simulink library "VLSGains"  (R2022b)
settings: Solver=VariableStepAuto  StartTime=0.0  StopTime=10.0  RelTol=1e-3
values from neighbouring files (symbols this model uses):
  VLSGainsConfig = struct('sample_rate_in_hertz', sample_rate_in_hertz,                              'frame_size', frame_size,                              'rgain_SILENT_GAIN', rgain_SILENT_GAIN,                              'granularity', internal_granularity,                              'numGains', numGains)    [VLSGainsInit.m]
  VLSGainsTune = load(VLSGainsTuneFileName)    [VLSGainsInit.m]
undefined symbols (not defined in the file or in its folder): Row
libraries: TuneVar x36, TOP x18, FeaturePath x2
(part 1 of 2)
settings Model: Creator=ud1041536  LastModifiedBy=jr1038734
settings SolverCC: AlgebraicLoopSolver=TrustRegion
settings DebuggingCC: UnconnectedInputMsg=warning  UnconnectedOutputMsg=warning  UnconnectedLineMsg=warning  SFMachineParentedDataDiag=warning
settings ModelReferenceCC: EnableRefExpFcnMdlSchedulingChecks=on

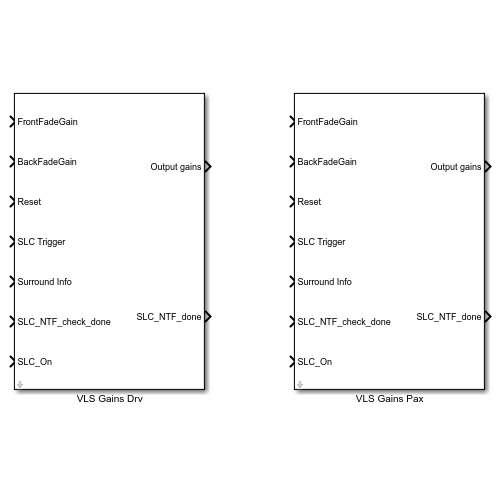
[thumbnail: Simulink's stored preview of the top-level diagram]
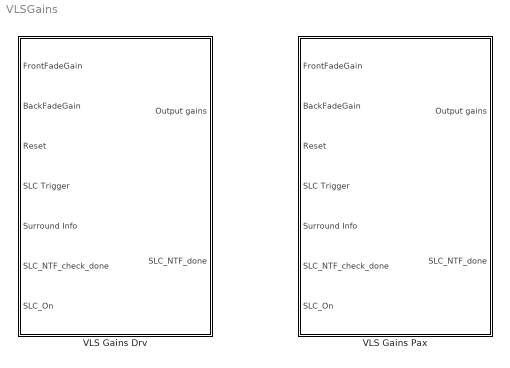
== system VLSGains ==
  VLS Gains Drv : Subsystem  mask(VLS Gains){configStruct=VLSGainsConfig, tuneStruct=VLSGainsTune, FeatureName=DrvGains}
      mask prompts: configStruct "Config struct name:"; tuneStruct "Tune struct name:"; FeatureName "FeaturePath name:"
      mask init:
      | VLSGainsMaskInit(gcbh, FeatureName);
      mask TypeOptions FeatureName: FeaturePath/FeatureName
  VLS Gains Pax : Subsystem  mask(VLS Gains){configStruct=VLSGainsConfig, tuneStruct=VLSGainsTune, FeatureName=PaxGains}
      mask prompts: configStruct "Config struct name:"; tuneStruct "Tune struct name:"; FeatureName "FeaturePath name:"
      mask init:
      | VLSGainsMaskInit(gcbh, FeatureName);
      mask TypeOptions FeatureName: FeaturePath/FeatureName

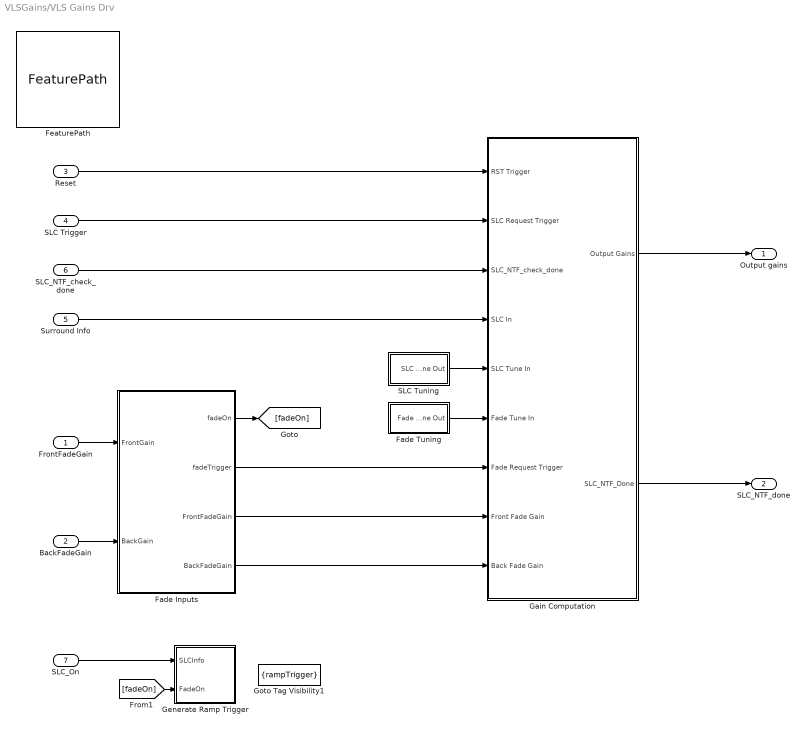
== system VLSGains/VLS Gains Drv ==
  FrontFadeGain : Inport
  BackFadeGain : Inport  Port=2
  Reset : Inport  Port=3
  SLC Trigger : Inport  Port=4
  Surround Info : Inport  Port=5
  SLC_NTF_check_done : Inport  Port=6
  SLC_On : Inport  Port=7
  Fade Inputs : Subsystem
  Fade Tuning : Subsystem
  FeaturePath : FeaturePath/FeaturePath  FeatureName=DrvGains  IsGroup=off  GroupNumber=-1  IsModule=off  TriggerInit=[125 254 250 371]
      settings: SourceProductName=Bose Talaria
  Gain Computation : Subsystem
  Generate Ramp Trigger : Subsystem
  Goto Tag Visibility1 : GotoTagVisibility  GotoTag=rampTrigger
  SLC Tuning : Subsystem
  Output gains : Outport  VectorParamsAs1DForOutWhenUnconnected=off
  SLC_NTF_done : Outport  Port=2  VectorParamsAs1DForOutWhenUnconnected=off
  wires:
  FrontFadeGain/1 -> Fade Inputs/1(FrontGain)
  Gain Computation/2(SLC_NTF_Done) -> SLC_NTF_done/1
  BackFadeGain/1 -> Fade Inputs/2(BackGain)
  SLC_NTF_check_done/1 -> Gain Computation/3(SLC_NTF_check_done)
  Reset/1 -> Gain Computation/1(RST Trigger)
  SLC Trigger/1 -> Gain Computation/2(SLC Request Trigger)
  Fade Tuning/1(Fade Tune Out) -> Gain Computation/6(Fade Tune In)
  Fade Inputs/3(FrontFadeGain) -> Gain Computation/8(Front Fade Gain)
  Gain Computation/1(Output Gains) -> Output gains/1
  Surround Info/1 -> Gain Computation/4(SLC In)
  Fade Inputs/4(BackFadeGain) -> Gain Computation/9(Back Fade Gain)
  SLC Tuning/1(SLC Tune Out) -> Gain Computation/5(SLC Tune In)
  Fade Inputs/2(fadeTrigger) -> Gain Computation/7(Fade Request Trigger)
  [fadeOn] -> Generate Ramp Trigger/2(FadeOn)
  SLC_On/1 -> Generate Ramp Trigger/1(SLCInfo)
  Fade Inputs/1(fadeOn) -> [fadeOn]

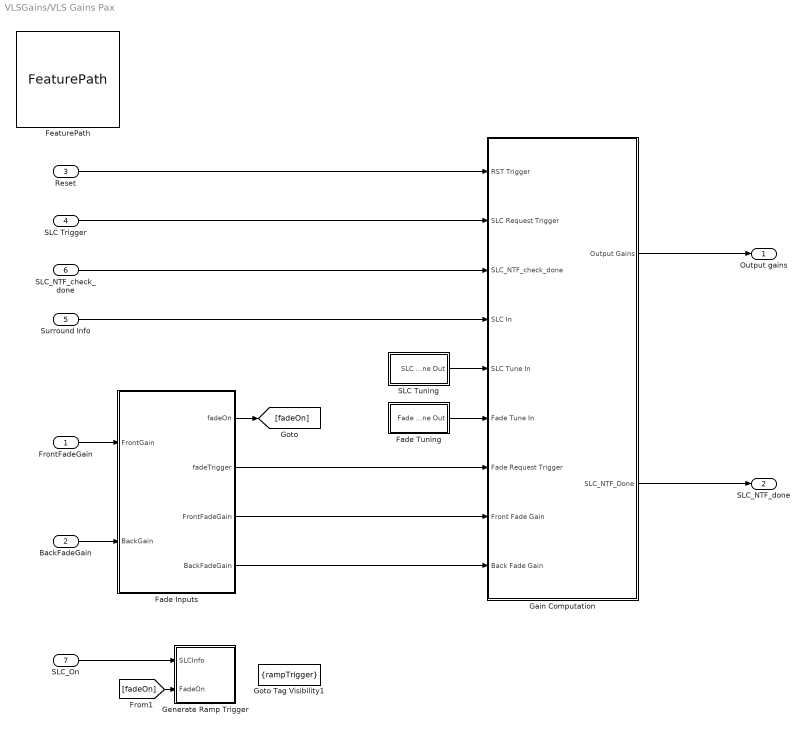
== system VLSGains/VLS Gains Pax ==
  FrontFadeGain : Inport
  BackFadeGain : Inport  Port=2
  Reset : Inport  Port=3
  SLC Trigger : Inport  Port=4
  Surround Info : Inport  Port=5
  SLC_NTF_check_done : Inport  Port=6
  SLC_On : Inport  Port=7
  Fade Inputs : Subsystem
  Fade Tuning : Subsystem
  FeaturePath : FeaturePath/FeaturePath  FeatureName=PaxGains  IsGroup=off  GroupNumber=-1  IsModule=off  TriggerInit=[125 254 250 371]
      settings: SourceProductName=Bose Talaria
  Gain Computation : Subsystem
  Generate Ramp Trigger : Subsystem
  Goto Tag Visibility1 : GotoTagVisibility  GotoTag=rampTrigger
  SLC Tuning : Subsystem
  Output gains : Outport  VectorParamsAs1DForOutWhenUnconnected=off
  SLC_NTF_done : Outport  Port=2  VectorParamsAs1DForOutWhenUnconnected=off
  wires:
  FrontFadeGain/1 -> Fade Inputs/1(FrontGain)
  Gain Computation/2(SLC_NTF_Done) -> SLC_NTF_done/1
  BackFadeGain/1 -> Fade Inputs/2(BackGain)
  SLC_NTF_check_done/1 -> Gain Computation/3(SLC_NTF_check_done)
  Reset/1 -> Gain Computation/1(RST Trigger)
  SLC Trigger/1 -> Gain Computation/2(SLC Request Trigger)
  Fade Tuning/1(Fade Tune Out) -> Gain Computation/6(Fade Tune In)
  Fade Inputs/3(FrontFadeGain) -> Gain Computation/8(Front Fade Gain)
  Gain Computation/1(Output Gains) -> Output gains/1
  Surround Info/1 -> Gain Computation/4(SLC In)
  Fade Inputs/4(BackFadeGain) -> Gain Computation/9(Back Fade Gain)
  SLC Tuning/1(SLC Tune Out) -> Gain Computation/5(SLC Tune In)
  Fade Inputs/2(fadeTrigger) -> Gain Computation/7(Fade Request Trigger)
  [fadeOn] -> Generate Ramp Trigger/2(FadeOn)
  SLC_On/1 -> Generate Ramp Trigger/1(SLCInfo)
  Fade Inputs/1(fadeOn) -> [fadeOn]

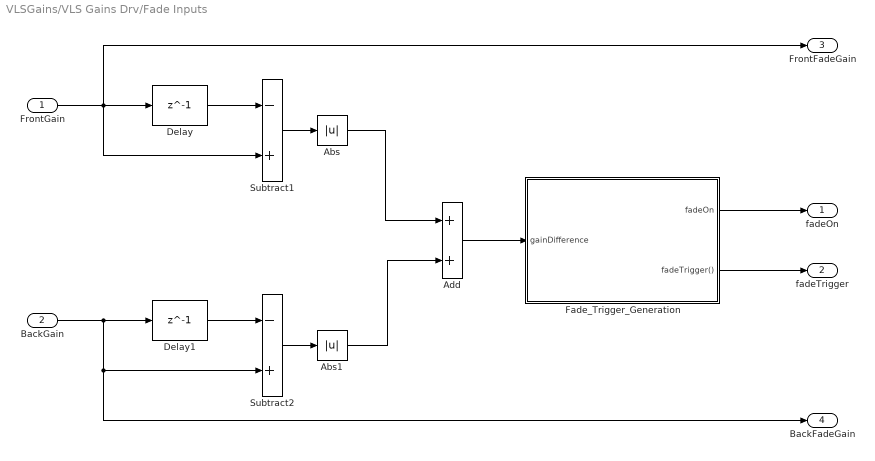
== system VLSGains/VLS Gains Drv/Fade Inputs ==
  FrontGain : Inport
  BackGain : Inport  Port=2
  Abs : Abs  SaturateOnIntegerOverflow=off
  Abs1 : Abs  SaturateOnIntegerOverflow=off
  Add : Sum
  Delay : Delay  DelayLength=1
  Delay1 : Delay  DelayLength=1
  Fade_Trigger_Generation : MATLAB Function  TreatAsAtomicUnit=on
  Subtract1 : Sum  Inputs=-+
  Subtract2 : Sum  Inputs=-+
  fadeOn : Outport
  fadeTrigger : Outport  Port=2  VectorParamsAs1DForOutWhenUnconnected=off
  FrontFadeGain : Outport  Port=3  VectorParamsAs1DForOutWhenUnconnected=off
  BackFadeGain : Outport  Port=4  VectorParamsAs1DForOutWhenUnconnected=off
  wires:
  BackGain/1 -> BackFadeGain/1, Subtract2/2, Delay1/1
  Abs1/1 -> Add/2
  Abs/1 -> Add/1
  Subtract2/1 -> Abs1/1
  Subtract1/1 -> Abs/1
  FrontGain/1 -> Subtract1/2, FrontFadeGain/1, Delay/1
  Delay/1 -> Subtract1/1
  Delay1/1 -> Subtract2/1
  Add/1 -> Fade_Trigger_Generation/1(gainDifference)
  Fade_Trigger_Generation/2(fadeTrigger()) -> fadeTrigger/1
  Fade_Trigger_Generation/1(fadeOn) -> fadeOn/1

== system VLSGains/VLS Gains Drv/Fade Tuning ==
  Backward Downmix Max : Subsystem  Description=This is the fraction of downmixing that occurs when 100% fade (back) is reached.
  Backward Downmix Threshold : Subsystem  Description=This is the fraction of fade (back) at which downmixing of premix coefficients starts.
  Downmix Weights : Subsystem  Description=These are the mixing weights at fader extreme when downmix_max is set to 1.
  Forward Downmix Threshold : Subsystem  Description=This is the fraction of fade (front) at which downmixing of premix coefficients starts.
  Foward Downmix Max : Subsystem  Description=This is the fraction of downmixing that occurs when 100% fade (front) is reached.
  Bus Element Out : Outport  VectorParamsAs1DForOutWhenUnconnected=off  PortName=Fade Tune Out  Element=Forward Downmix Threshold
  Bus Element Out1 : Outport  VectorParamsAs1DForOutWhenUnconnected=off  PortName=Fade Tune Out  Element=Forward Downmix Max
  Bus Element Out2 : Outport  VectorParamsAs1DForOutWhenUnconnected=off  PortName=Fade Tune Out  Element=Backward Downmix Threshold
  Bus Element Out3 : Outport  VectorParamsAs1DForOutWhenUnconnected=off  PortName=Fade Tune Out  Element=Backward Downmix Max
  Bus Element Out4 : Outport  VectorParamsAs1DForOutWhenUnconnected=off  PortName=Fade Tune Out  Element=Downmix Weights
  wires:
  Downmix Weights/1(Out1) -> Bus Element Out4/1
  Backward Downmix Threshold/1(Out1) -> Bus Element Out2/1
  Backward Downmix Max/1(Out1) -> Bus Element Out3/1
  Foward Downmix Max/1(Out1) -> Bus Element Out1/1
  Forward Downmix Threshold/1(Out1) -> Bus Element Out/1

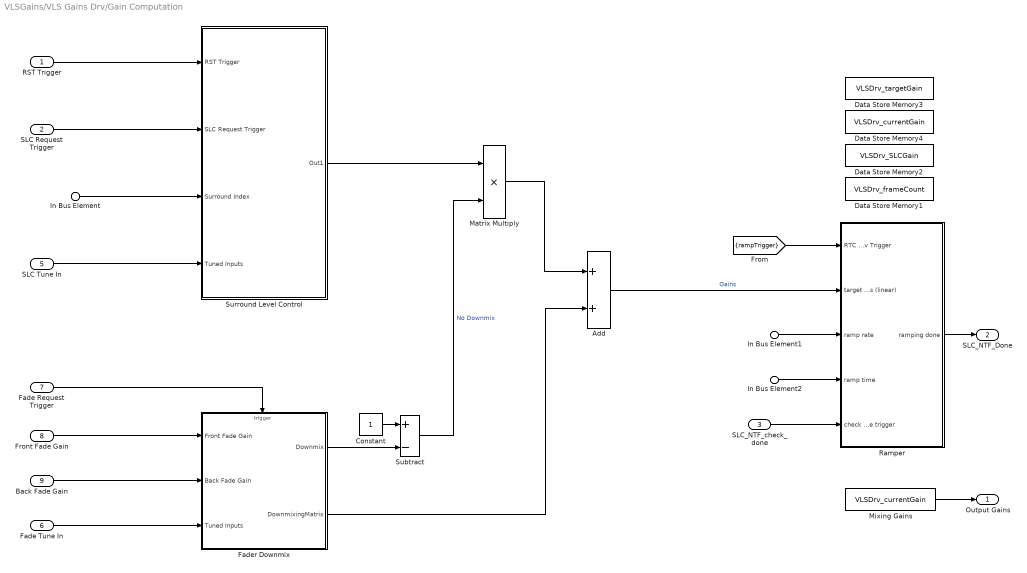
== system VLSGains/VLS Gains Drv/Gain Computation ==
  RST Trigger : Inport
  SLC Request Trigger : Inport  Port=2
  SLC_NTF_check_done : Inport  Port=3
  In Bus Element : Inport  Port=4  PortName=SLC In  Element=surround_index
  In Bus Element1 : Inport  Port=4  PortName=SLC In  Element=ramp_db_per_second
  In Bus Element2 : Inport  Port=4  PortName=SLC In  Element=ramp_milliseconds
  SLC Tune In : Inport  Port=5
  Fade Tune In : Inport  Port=6
  Fade Request Trigger : Inport  Port=7
  Front Fade Gain : Inport  Port=8
  Back Fade Gain : Inport  Port=9
  Add : Sum
  Constant : Constant  OutDataTypeStr=single
  Data Store Memory1 : DataStoreMemory  DataStoreName=VLSDrv_frameCount  ReadBeforeWriteMsg=warning  WriteAfterWriteMsg=warning  WriteAfterReadMsg=warning  InitialValue=zeros(configStruct.numGains,1)  ShowAdditionalParam=off  OutDataTypeStr=int32
  Data Store Memory2 : DataStoreMemory  DataStoreName=VLSDrv_SLCGain  ReadBeforeWriteMsg=warning  WriteAfterWriteMsg=warning  WriteAfterReadMsg=warning  InitialValue=1e-5*ones(configStruct.numGains,1)  ShowAdditionalParam=off  OutDataTypeStr=single
  Data Store Memory3 : DataStoreMemory  DataStoreName=VLSDrv_targetGain  ReadBeforeWriteMsg=warning  WriteAfterWriteMsg=warning  WriteAfterReadMsg=warning  InitialValue=1e-5*ones(configStruct.numGains,1)  ShowAdditionalParam=off  OutDataTypeStr=single
  Data Store Memory4 : DataStoreMemory  DataStoreName=VLSDrv_currentGain  ReadBeforeWriteMsg=warning  WriteAfterWriteMsg=warning  WriteAfterReadMsg=warning  InitialValue=1e-5*ones(configStruct.numGains,1)  ShowAdditionalParam=off  OutDataTypeStr=single
  Fader Downmix : Subsystem
  Matrix Multiply : Product
  Mixing Gains : DataStoreRead  DataStoreName=VLSDrv_currentGain  IndexOptions=Index vector (dialog)  Indices=1  OutputSizes=1
  Ramper : Subsystem
  Subtract : Sum  Inputs=+-
  Surround Level Control : Subsystem
  Output Gains : Outport
  SLC_NTF_Done : Outport  Port=2  VectorParamsAs1DForOutWhenUnconnected=off
  wires:
  Constant/1 -> Subtract/1
  Subtract/1 -> Matrix Multiply/2  "No Downmix"
  Fader Downmix/2(DownmixingMatrix) -> Add/2
  Fade Request Trigger/1 -> Fader Downmix/Trigger
  RST Trigger/1 -> Surround Level Control/1(RST Trigger)
  Back Fade Gain/1 -> Fader Downmix/2(Back Fade Gain)
  SLC Request Trigger/1 -> Surround Level Control/2(SLC Request Trigger)
  In Bus Element/1 -> Surround Level Control/3(Surround Index)
  Fader Downmix/1(Downmix) -> Subtract/2
  Fade Tune In/1 -> Fader Downmix/3(Tuned Inputs)
  Matrix Multiply/1 -> Add/1
  SLC Tune In/1 -> Surround Level Control/4(Tuned Inputs)
  Add/1 -> Ramper/2(target gains (linear))  "Gains"
  Front Fade Gain/1 -> Fader Downmix/1(Front Fade Gain)
  Surround Level Control/1(Out1) -> Matrix Multiply/1
  SLC_NTF_check_done/1 -> Ramper/5(check sequence trigger)
  [rampTrigger] -> Ramper/1(RTC Recv Trigger)
  Ramper/1(ramping done) -> SLC_NTF_Done/1
  Mixing Gains/1 -> Output Gains/1
  In Bus Element2/1 -> Ramper/4(ramp time)
  In Bus Element1/1 -> Ramper/3(ramp rate)

== system VLSGains/VLS Gains Drv/Generate Ramp Trigger ==
  SLCInfo : Inport
  FadeOn : Inport  Port=2
  MATLAB Function : MATLAB Function  TreatAsAtomicUnit=on
  Terminator : Terminator
  tag scope: rampTrigger=scoped
  wires:
  MATLAB Function/2(ramp()) -> [rampTrigger]
  FadeOn/1 -> MATLAB Function/2(Fade_On)
  SLCInfo/1 -> MATLAB Function/1(SLC_On)
  MATLAB Function/1(rampOn) -> Terminator/1

== system VLSGains/VLS Gains Drv/SLC Tuning ==
  Detent Level : Subsystem  Description="This is the premix (scalar mixing) matrix for the detent (default) level of \"surroundiness\"."
  Interpolation Method : Subsystem  Description=|
      | This controls the method used to interpolate premix coefficient matrix as the surround knob is adjusted.
      | - 0 for linear interpolation (default)
      | - 1 for db-linear interpolation
  Max Level : Subsystem  Description="This is the premix (scalar mixing) matrix for the maximum level of \"surroundiness\"."
  Min Level : Subsystem  Description="This is the premix (scalar mixing) matrix for the minimum level of \"surroundiness\" i.e. steroe case."
  Bus Element Out : Outport  VectorParamsAs1DForOutWhenUnconnected=off  PortName=SLC Tune Out  Element=Interpolation Method
  Bus Element Out1 : Outport  VectorParamsAs1DForOutWhenUnconnected=off  PortName=SLC Tune Out  Element=Min Level
  Bus Element Out2 : Outport  VectorParamsAs1DForOutWhenUnconnected=off  PortName=SLC Tune Out  Element=Detent Level
  Bus Element Out3 : Outport  VectorParamsAs1DForOutWhenUnconnected=off  PortName=SLC Tune Out  Element=Max Level
  wires:
  Max Level/1(Out1) -> Bus Element Out3/1
  Detent Level/1(Out1) -> Bus Element Out2/1
  Min Level/1(Out1) -> Bus Element Out1/1
  Interpolation Method/1(Out1) -> Bus Element Out/1

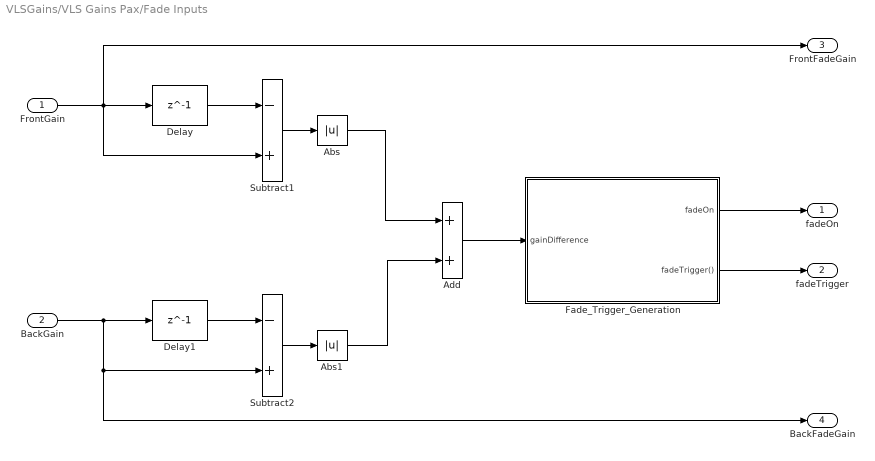
== system VLSGains/VLS Gains Pax/Fade Inputs ==
  FrontGain : Inport
  BackGain : Inport  Port=2
  Abs : Abs  SaturateOnIntegerOverflow=off
  Abs1 : Abs  SaturateOnIntegerOverflow=off
  Add : Sum
  Delay : Delay  DelayLength=1
  Delay1 : Delay  DelayLength=1
  Fade_Trigger_Generation : MATLAB Function  TreatAsAtomicUnit=on
  Subtract1 : Sum  Inputs=-+
  Subtract2 : Sum  Inputs=-+
  fadeOn : Outport
  fadeTrigger : Outport  Port=2  VectorParamsAs1DForOutWhenUnconnected=off
  FrontFadeGain : Outport  Port=3  VectorParamsAs1DForOutWhenUnconnected=off
  BackFadeGain : Outport  Port=4  VectorParamsAs1DForOutWhenUnconnected=off
  wires:
  BackGain/1 -> BackFadeGain/1, Subtract2/2, Delay1/1
  Abs1/1 -> Add/2
  Abs/1 -> Add/1
  Subtract2/1 -> Abs1/1
  Subtract1/1 -> Abs/1
  FrontGain/1 -> Subtract1/2, FrontFadeGain/1, Delay/1
  Delay/1 -> Subtract1/1
  Delay1/1 -> Subtract2/1
  Add/1 -> Fade_Trigger_Generation/1(gainDifference)
  Fade_Trigger_Generation/2(fadeTrigger()) -> fadeTrigger/1
  Fade_Trigger_Generation/1(fadeOn) -> fadeOn/1

== system VLSGains/VLS Gains Pax/Fade Tuning ==
  Backward Downmix Max : Subsystem  Description=This is the fraction of downmixing that occurs when 100% fade (back) is reached.
  Backward Downmix Threshold : Subsystem  Description=This is the fraction of fade (back) at which downmixing of premix coefficients starts.
  Downmix Weights : Subsystem  Description=These are the mixing weights at fader extreme when downmix_max is set to 1.
  Forward Downmix Threshold : Subsystem  Description=This is the fraction of fade (front) at which downmixing of premix coefficients starts.
  Foward Downmix Max : Subsystem  Description=This is the fraction of downmixing that occurs when 100% fade (front) is reached.
  Bus Element Out : Outport  VectorParamsAs1DForOutWhenUnconnected=off  PortName=Fade Tune Out  Element=Forward Downmix Threshold
  Bus Element Out1 : Outport  VectorParamsAs1DForOutWhenUnconnected=off  PortName=Fade Tune Out  Element=Forward Downmix Max
  Bus Element Out2 : Outport  VectorParamsAs1DForOutWhenUnconnected=off  PortName=Fade Tune Out  Element=Backward Downmix Threshold
  Bus Element Out3 : Outport  VectorParamsAs1DForOutWhenUnconnected=off  PortName=Fade Tune Out  Element=Backward Downmix Max
  Bus Element Out4 : Outport  VectorParamsAs1DForOutWhenUnconnected=off  PortName=Fade Tune Out  Element=Downmix Weights
  wires:
  Downmix Weights/1(Out1) -> Bus Element Out4/1
  Backward Downmix Threshold/1(Out1) -> Bus Element Out2/1
  Backward Downmix Max/1(Out1) -> Bus Element Out3/1
  Foward Downmix Max/1(Out1) -> Bus Element Out1/1
  Forward Downmix Threshold/1(Out1) -> Bus Element Out/1

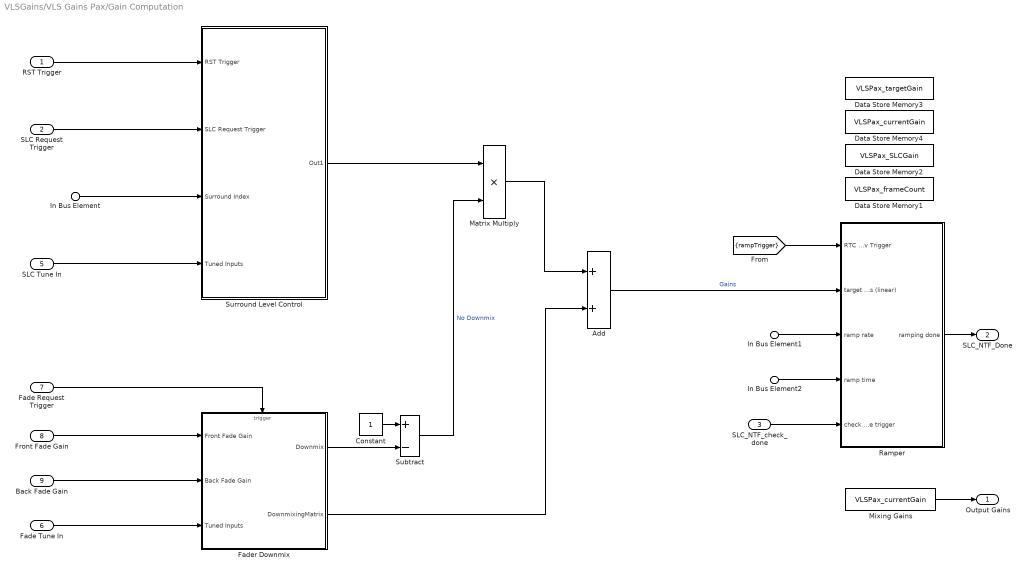
== system VLSGains/VLS Gains Pax/Gain Computation ==
  RST Trigger : Inport
  SLC Request Trigger : Inport  Port=2
  SLC_NTF_check_done : Inport  Port=3
  In Bus Element : Inport  Port=4  PortName=SLC In  Element=surround_index
  In Bus Element1 : Inport  Port=4  PortName=SLC In  Element=ramp_db_per_second
  In Bus Element2 : Inport  Port=4  PortName=SLC In  Element=ramp_milliseconds
  SLC Tune In : Inport  Port=5
  Fade Tune In : Inport  Port=6
  Fade Request Trigger : Inport  Port=7
  Front Fade Gain : Inport  Port=8
  Back Fade Gain : Inport  Port=9
  Add : Sum
  Constant : Constant  OutDataTypeStr=single
  Data Store Memory1 : DataStoreMemory  DataStoreName=VLSPax_frameCount  ReadBeforeWriteMsg=warning  WriteAfterWriteMsg=warning  WriteAfterReadMsg=warning  InitialValue=zeros(configStruct.numGains,1)  ShowAdditionalParam=off  OutDataTypeStr=int32
  Data Store Memory2 : DataStoreMemory  DataStoreName=VLSPax_SLCGain  ReadBeforeWriteMsg=warning  WriteAfterWriteMsg=warning  WriteAfterReadMsg=warning  InitialValue=1e-5*ones(configStruct.numGains,1)  ShowAdditionalParam=off  OutDataTypeStr=single
  Data Store Memory3 : DataStoreMemory  DataStoreName=VLSPax_targetGain  ReadBeforeWriteMsg=warning  WriteAfterWriteMsg=warning  WriteAfterReadMsg=warning  InitialValue=1e-5*ones(configStruct.numGains,1)  ShowAdditionalParam=off  OutDataTypeStr=single
  Data Store Memory4 : DataStoreMemory  DataStoreName=VLSPax_currentGain  ReadBeforeWriteMsg=warning  WriteAfterWriteMsg=warning  WriteAfterReadMsg=warning  InitialValue=1e-5*ones(configStruct.numGains,1)  ShowAdditionalParam=off  OutDataTypeStr=single
  Fader Downmix : Subsystem
  Matrix Multiply : Product
  Mixing Gains : DataStoreRead  DataStoreName=VLSPax_currentGain  IndexOptions=Index vector (dialog)  Indices=1  OutputSizes=1
  Ramper : Subsystem
  Subtract : Sum  Inputs=+-
  Surround Level Control : Subsystem
  Output Gains : Outport
  SLC_NTF_Done : Outport  Port=2  VectorParamsAs1DForOutWhenUnconnected=off
  wires:
  Constant/1 -> Subtract/1
  Subtract/1 -> Matrix Multiply/2  "No Downmix"
  Fader Downmix/2(DownmixingMatrix) -> Add/2
  Fade Request Trigger/1 -> Fader Downmix/Trigger
  RST Trigger/1 -> Surround Level Control/1(RST Trigger)
  Back Fade Gain/1 -> Fader Downmix/2(Back Fade Gain)
  SLC Request Trigger/1 -> Surround Level Control/2(SLC Request Trigger)
  In Bus Element/1 -> Surround Level Control/3(Surround Index)
  Fader Downmix/1(Downmix) -> Subtract/2
  Fade Tune In/1 -> Fader Downmix/3(Tuned Inputs)
  Matrix Multiply/1 -> Add/1
  SLC Tune In/1 -> Surround Level Control/4(Tuned Inputs)
  Add/1 -> Ramper/2(target gains (linear))  "Gains"
  Front Fade Gain/1 -> Fader Downmix/1(Front Fade Gain)
  Surround Level Control/1(Out1) -> Matrix Multiply/1
  SLC_NTF_check_done/1 -> Ramper/5(check sequence trigger)
  [rampTrigger] -> Ramper/1(RTC Recv Trigger)
  Ramper/1(ramping done) -> SLC_NTF_Done/1
  Mixing Gains/1 -> Output Gains/1
  In Bus Element2/1 -> Ramper/4(ramp time)
  In Bus Element1/1 -> Ramper/3(ramp rate)

== system VLSGains/VLS Gains Pax/Generate Ramp Trigger ==
  SLCInfo : Inport
  FadeOn : Inport  Port=2
  MATLAB Function : MATLAB Function  TreatAsAtomicUnit=on
  Terminator : Terminator
  tag scope: rampTrigger=scoped
  wires:
  MATLAB Function/2(ramp()) -> [rampTrigger]
  FadeOn/1 -> MATLAB Function/2(Fade_On)
  SLCInfo/1 -> MATLAB Function/1(SLC_On)
  MATLAB Function/1(rampOn) -> Terminator/1

== system VLSGains/VLS Gains Pax/SLC Tuning ==
  Detent Level : Subsystem  Description="This is the premix (scalar mixing) matrix for the detent (default) level of \"surroundiness\"."
  Interpolation Method : Subsystem  Description=|
      | This controls the method used to interpolate premix coefficient matrix as the surround knob is adjusted.
      | - 0 for linear interpolation (default)
      | - 1 for db-linear interpolation
  Max Level : Subsystem  Description="This is the premix (scalar mixing) matrix for the maximum level of \"surroundiness\"."
  Min Level : Subsystem  Description="This is the premix (scalar mixing) matrix for the minimum level of \"surroundiness\" i.e. steroe case."
  Bus Element Out : Outport  VectorParamsAs1DForOutWhenUnconnected=off  PortName=SLC Tune Out  Element=Interpolation Method
  Bus Element Out1 : Outport  VectorParamsAs1DForOutWhenUnconnected=off  PortName=SLC Tune Out  Element=Min Level
  Bus Element Out2 : Outport  VectorParamsAs1DForOutWhenUnconnected=off  PortName=SLC Tune Out  Element=Detent Level
  Bus Element Out3 : Outport  VectorParamsAs1DForOutWhenUnconnected=off  PortName=SLC Tune Out  Element=Max Level
  wires:
  Max Level/1(Out1) -> Bus Element Out3/1
  Detent Level/1(Out1) -> Bus Element Out2/1
  Min Level/1(Out1) -> Bus Element Out1/1
  Interpolation Method/1(Out1) -> Bus Element Out/1

== system VLSGains/VLS Gains Drv/Fade Tuning/Backward Downmix Max ==
  TOP : TOP/TOP  TriggerInit=[440 20 585 80]  TopName=BackwardDownmixMax  DataType=single  BankNumber=0  PreOverlay=false  PostOverlay=false  Role=Automatic
      settings: SourceProductName=Bose Talaria
  TranslateTrigger : TuneVar/TranslateTrigger  TriggerInit=[286 -100 324 -45]
      settings: SourceProductName=Bose Talaria
  Trivial Translation : MATLAB Function  TreatAsAtomicUnit=on
  Tune Variable : TuneVar/TuneVar  TuneName=BackwardDownmixMax  SpecifyMaxSize=off  VariableDim=1 (Row)  MaxSize=[1 1]  TunabilityNumber=1  MinValue=[0]  MaxValue=[1]  TriggerInit=[-65 25 105 75]  MaskValue=tuneStruct.BackwardDownmixMax
      settings: SourceProductName=Bose Talaria
  Out1 : Outport  VectorParamsAs1DForOutWhenUnconnected=off
  wires:
  TranslateTrigger/1 -> Trivial Translation/Trigger
  Trivial Translation/1(TOP) -> TOP/1
  Tune Variable/1 -> Trivial Translation/1(BackwardDownmixMax)  "BackwardDownmixMax"
  TOP/1 -> Out1/1  "BackwardDownmixMax"

== system VLSGains/VLS Gains Drv/Fade Tuning/Backward Downmix Threshold ==
  TOP : TOP/TOP  TriggerInit=[440 20 585 80]  TopName=BackwardDownmixThreshold  DataType=single  BankNumber=0  PreOverlay=false  PostOverlay=false  Role=Automatic
      settings: SourceProductName=Bose Talaria
  TranslateTrigger : TuneVar/TranslateTrigger  TriggerInit=[306 -100 344 -45]
      settings: SourceProductName=Bose Talaria
  Trivial Translation : MATLAB Function  TreatAsAtomicUnit=on
  Tune Variable : TuneVar/TuneVar  TuneName=BackwardDownmixThreshold  SpecifyMaxSize=off  VariableDim=1 (Row)  MaxSize=[1 1]  TunabilityNumber=1  MinValue=[0]  MaxValue=[1]  TriggerInit=[-75 25 95 75]  MaskValue=tuneStruct.BackwardDownmixThreshold
      settings: SourceProductName=Bose Talaria
  Out1 : Outport  VectorParamsAs1DForOutWhenUnconnected=off
  wires:
  TranslateTrigger/1 -> Trivial Translation/Trigger
  Trivial Translation/1(TOP) -> TOP/1
  Tune Variable/1 -> Trivial Translation/1(BackwardDownmixThreshold)  "BackwardDownmixThreshold"
  TOP/1 -> Out1/1  "BackwardDownmixThreshold"

== system VLSGains/VLS Gains Drv/Fade Tuning/Downmix Weights ==
  TOP : TOP/TOP  TriggerInit=[385 17 610 83]  TopName=DownmixWeights  DataType=single  BankNumber=0  PreOverlay=false  PostOverlay=false  Role=Automatic
      settings: SourceProductName=Bose Talaria
  TranslateTrigger : TuneVar/TranslateTrigger  TriggerInit=[266 -100 304 -45]
      settings: SourceProductName=Bose Talaria
  Trivial Translation : MATLAB Function  TreatAsAtomicUnit=on
  Tune Variable : TuneVar/TuneVar  TuneName=DownmixWeights  SpecifyMaxSize=off  VariableDim=1 (Row)  MaxSize=[1 1]  TunabilityNumber=1  MinValue=[0]  MaxValue=[1]  TriggerInit=[-80 25 150 75]  MaskValue=tuneStruct.downmix_wts
      settings: SourceProductName=Bose Talaria
  Out1 : Outport  VectorParamsAs1DForOutWhenUnconnected=off
  wires:
  TranslateTrigger/1 -> Trivial Translation/Trigger
  Trivial Translation/1(TOP) -> TOP/1
  Tune Variable/1 -> Trivial Translation/1(downmix_wts)  "DownmixWeights"
  TOP/1 -> Out1/1  "DownmixWeights"

== system VLSGains/VLS Gains Drv/Fade Tuning/Forward Downmix Threshold ==
  TOP : TOP/TOP  TriggerInit=[440 20 585 80]  TopName=ForwardDownmixThreshold  DataType=single  BankNumber=0  PreOverlay=false  PostOverlay=false  Role=Automatic
      settings: SourceProductName=Bose Talaria
  TranslateTrigger : TuneVar/TranslateTrigger  TriggerInit=[291 -100 329 -45]
      settings: SourceProductName=Bose Talaria
  Trivial Translation : MATLAB Function  TreatAsAtomicUnit=on
  Tune Variable : TuneVar/TuneVar  TuneName=ForwardDownmixThreshold  SpecifyMaxSize=off  VariableDim=1 (Row)  MaxSize=[1 1]  TunabilityNumber=1  MinValue=[0]  MaxValue=[1]  TriggerInit=[-80 25 90 75]  MaskValue=tuneStruct.ForwardDownmixThreshold
      settings: SourceProductName=Bose Talaria
  Out1 : Outport  VectorParamsAs1DForOutWhenUnconnected=off
  wires:
  TranslateTrigger/1 -> Trivial Translation/Trigger
  Trivial Translation/1(TOP) -> TOP/1
  Tune Variable/1 -> Trivial Translation/1(ForwardDownmixThreshold)  "ForwardDownmixThreshold"
  TOP/1 -> Out1/1  "ForwardDownmixThreshold"

== system VLSGains/VLS Gains Drv/Fade Tuning/Foward Downmix Max ==
  TOP : TOP/TOP  TriggerInit=[440 20 585 80]  TopName=ForwardDownmixMax  DataType=single  BankNumber=0  PreOverlay=false  PostOverlay=false  Role=Automatic
      settings: SourceProductName=Bose Talaria
  TranslateTrigger : TuneVar/TranslateTrigger  TriggerInit=[286 -100 324 -45]
      settings: SourceProductName=Bose Talaria
  Trivial Translation : MATLAB Function  TreatAsAtomicUnit=on
  Tune Variable : TuneVar/TuneVar  TuneName=ForwardDownmixMax  SpecifyMaxSize=off  VariableDim=1 (Row)  MaxSize=[1 1]  TunabilityNumber=1  MinValue=[0]  MaxValue=[1]  TriggerInit=[-70 25 100 75]  MaskValue=tuneStruct.ForwardDownmixMax
      settings: SourceProductName=Bose Talaria
  Out1 : Outport  VectorParamsAs1DForOutWhenUnconnected=off
  wires:
  TranslateTrigger/1 -> Trivial Translation/Trigger
  Trivial Translation/1(TOP) -> TOP/1
  Tune Variable/1 -> Trivial Translation/1(ForwardDownmixMax)  "ForwardDownmixMax"
  TOP/1 -> Out1/1  "ForwardDownmixMax"

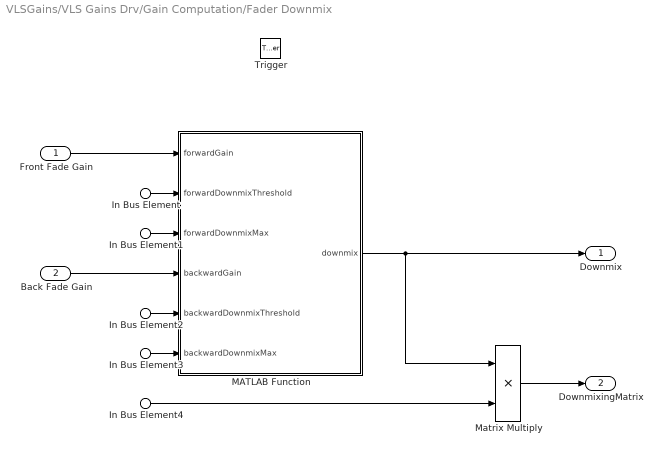
== system VLSGains/VLS Gains Drv/Gain Computation/Fader Downmix ==
  Front Fade Gain : Inport
  Back Fade Gain : Inport  Port=2
  In Bus Element : Inport  Port=3  PortName=Tuned Inputs  Element=Forward Downmix Threshold
  In Bus Element1 : Inport  Port=3  PortName=Tuned Inputs  Element=Forward Downmix Max
  In Bus Element2 : Inport  Port=3  PortName=Tuned Inputs  Element=Backward Downmix Threshold
  In Bus Element3 : Inport  Port=3  PortName=Tuned Inputs  Element=Backward Downmix Max
  In Bus Element4 : Inport  Port=3  PortName=Tuned Inputs  Element=Downmix Weights
  Trigger : TriggerPort  TriggerType=function-call  VariantControl=Variant  PortDimensions=1
  MATLAB Function : MATLAB Function  TreatAsAtomicUnit=on
  Matrix Multiply : Product
  Downmix : Outport  VectorParamsAs1DForOutWhenUnconnected=off
  DownmixingMatrix : Outport  Port=2  VectorParamsAs1DForOutWhenUnconnected=off
  wires:
  In Bus Element4/1 -> Matrix Multiply/2
  Matrix Multiply/1 -> DownmixingMatrix/1
  Back Fade Gain/1 -> MATLAB Function/4(backwardGain)
  Front Fade Gain/1 -> MATLAB Function/1(forwardGain)
  In Bus Element/1 -> MATLAB Function/2(forwardDownmixThreshold)
  In Bus Element1/1 -> MATLAB Function/3(forwardDownmixMax)
  In Bus Element2/1 -> MATLAB Function/5(backwardDownmixThreshold)
  In Bus Element3/1 -> MATLAB Function/6(backwardDownmixMax)
  MATLAB Function/1(downmix) -> Matrix Multiply/1, Downmix/1

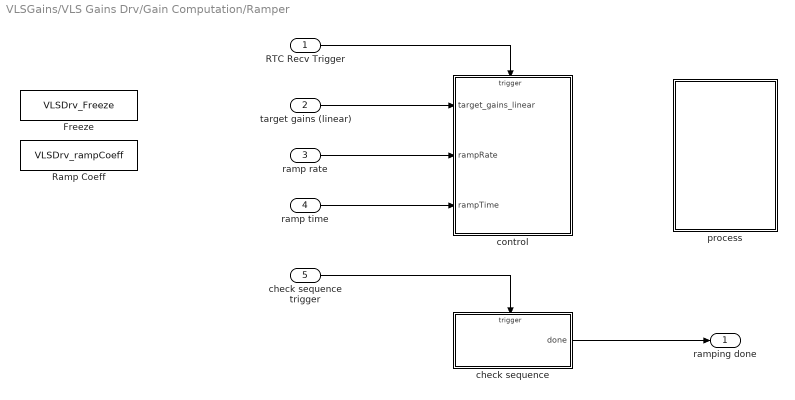
== system VLSGains/VLS Gains Drv/Gain Computation/Ramper ==
  RTC Recv Trigger : Inport
  target gains (linear) : Inport  Port=2
  ramp rate : Inport  Port=3
  ramp time : Inport  Port=4
  check sequence trigger : Inport  Port=5
  Freeze : DataStoreMemory  DataStoreName=VLSDrv_Freeze  ReadBeforeWriteMsg=warning  WriteAfterWriteMsg=warning  WriteAfterReadMsg=warning  ShowAdditionalParam=off  OutDataTypeStr=boolean
  Ramp Coeff : DataStoreMemory  DataStoreName=VLSDrv_rampCoeff  ReadBeforeWriteMsg=warning  WriteAfterWriteMsg=warning  WriteAfterReadMsg=warning  InitialValue=ones(configStruct.numGains,1)  ShowAdditionalParam=off  OutDataTypeStr=single
  check sequence : MATLAB Function  TreatAsAtomicUnit=on
  control : MATLAB Function  TreatAsAtomicUnit=on
  process : MATLAB Function  TreatAsAtomicUnit=on
  ramping done : Outport  VectorParamsAs1DForOutWhenUnconnected=off
  wires:
  target gains (linear)/1 -> control/1(target_gains_linear)
  RTC Recv Trigger/1 -> control/Trigger
  check sequence/1(done) -> ramping done/1
  check sequence trigger/1 -> check sequence/Trigger
  ramp time/1 -> control/3(rampTime)
  ramp rate/1 -> control/2(rampRate)

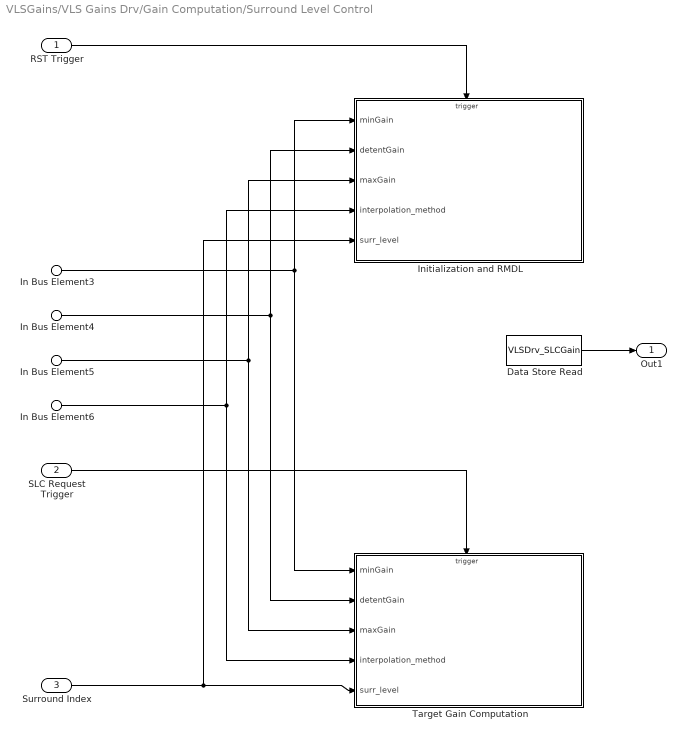
== system VLSGains/VLS Gains Drv/Gain Computation/Surround Level Control ==
  RST Trigger : Inport
  SLC Request Trigger : Inport  Port=2
  Surround Index : Inport  Port=3
  In Bus Element3 : Inport  Port=4  PortName=Tuned Inputs  Element=Min Level
  In Bus Element4 : Inport  Port=4  PortName=Tuned Inputs  Element=Detent Level
  In Bus Element5 : Inport  Port=4  PortName=Tuned Inputs  Element=Max Level
  In Bus Element6 : Inport  Port=4  PortName=Tuned Inputs  Element=Interpolation Method
  Data Store Read : DataStoreRead  DataStoreName=VLSDrv_SLCGain  IndexOptions=Index vector (dialog)  Indices=1  OutputSizes=1
  Initialization and RMDL : MATLAB Function  TreatAsAtomicUnit=on
  Target Gain Computation : MATLAB Function  TreatAsAtomicUnit=on
  Out1 : Outport
  wires:
  In Bus Element4/1 -> Target Gain Computation/2(detentGain), Initialization and RMDL/2(detentGain)
  In Bus Element3/1 -> Initialization and RMDL/1(minGain), Target Gain Computation/1(minGain)
  In Bus Element6/1 -> Initialization and RMDL/4(interpolation_method), Target Gain Computation/4(interpolation_method)
  In Bus Element5/1 -> Initialization and RMDL/3(maxGain), Target Gain Computation/3(maxGain)
  SLC Request Trigger/1 -> Target Gain Computation/Trigger
  RST Trigger/1 -> Initialization and RMDL/Trigger
  Surround Index/1 -> Initialization and RMDL/5(surr_level), Target Gain Computation/5(surr_level)
  Data Store Read/1 -> Out1/1

== system VLSGains/VLS Gains Drv/SLC Tuning/Detent Level ==
  TOP : TOP/TOP  TriggerInit=[405 22 635 78]  TopName=DetentLevel  DataType=single  BankNumber=0  PreOverlay=false  PostOverlay=false  Role=Automatic
      settings: SourceProductName=Bose Talaria
  TranslateTrigger : TuneVar/TranslateTrigger  TriggerInit=[266 -100 304 -45]
      settings: SourceProductName=Bose Talaria
  Trivial Translation : MATLAB Function  TreatAsAtomicUnit=on
  Tune Variable : TuneVar/TuneVar  TuneName=DetentLevel  SpecifyMaxSize=off  VariableDim=1 (Row)  MaxSize=[1 1]  TunabilityNumber=1  MinValue=[0]  MaxValue=[1]  TriggerInit=[-110 25 105 75]  MaskValue=tuneStruct.detentGain
      settings: SourceProductName=Bose Talaria
  Out1 : Outport  VectorParamsAs1DForOutWhenUnconnected=off
  wires:
  TranslateTrigger/1 -> Trivial Translation/Trigger
  Trivial Translation/1(TOP) -> TOP/1
  Tune Variable/1 -> Trivial Translation/1(detentGain)  "DetentLevel"
  TOP/1 -> Out1/1  "DetentLevel"

== system VLSGains/VLS Gains Drv/SLC Tuning/Interpolation Method ==
  TOP : TOP/TOP  TriggerInit=[440 20 585 80]  TopName=Interpolation_Method  DataType=single  BankNumber=0  PreOverlay=false  PostOverlay=false  Role=Automatic
      settings: SourceProductName=Bose Talaria
  TranslateTrigger : TuneVar/TranslateTrigger  TriggerInit=[306 -100 344 -45]
      settings: SourceProductName=Bose Talaria
  Trivial Translation : MATLAB Function  TreatAsAtomicUnit=on
  Tune Variable : TuneVar/TuneVar  TuneName=Interpolation_Method  SpecifyMaxSize=off  VariableDim=1 (Row)  MaxSize=[1 1]  TunabilityNumber=2  MinValue=[0]  MaxValue=[1]  TriggerInit=[-40 25 130 75]  MaskValue=tuneStruct.interpolationMethod
      settings: SourceProductName=Bose Talaria
  Out1 : Outport  VectorParamsAs1DForOutWhenUnconnected=off
  wires:
  TranslateTrigger/1 -> Trivial Translation/Trigger
  Trivial Translation/1(TOP) -> TOP/1
  Tune Variable/1 -> Trivial Translation/1(interpolationMethod)  "Interpolation_Method"
  TOP/1 -> Out1/1  "Interpolation_Method"

== system VLSGains/VLS Gains Drv/SLC Tuning/Max Level ==
  TOP : TOP/TOP  TriggerInit=[425 22 630 78]  TopName=MaxLevel  DataType=single  BankNumber=0  PreOverlay=false  PostOverlay=false  Role=Automatic
      settings: SourceProductName=Bose Talaria
  TranslateTrigger : TuneVar/TranslateTrigger  TriggerInit=[306 -100 344 -45]
      settings: SourceProductName=Bose Talaria
  Trivial Translation : MATLAB Function  TreatAsAtomicUnit=on
  Tune Variable : TuneVar/TuneVar  TuneName=MaxLevel  SpecifyMaxSize=off  VariableDim=1 (Row)  MaxSize=[1 1]  TunabilityNumber=1  MinValue=[0]  MaxValue=[1]  TriggerInit=[-55 25 145 75]  MaskValue=tuneStruct.maxGain
      settings: SourceProductName=Bose Talaria
  Out1 : Outport  VectorParamsAs1DForOutWhenUnconnected=off
  wires:
  TranslateTrigger/1 -> Trivial Translation/Trigger
  Trivial Translation/1(TOP) -> TOP/1
  Tune Variable/1 -> Trivial Translation/1(maxGain)  "MaxLevel"
  TOP/1 -> Out1/1  "MaxLevel"

== system VLSGains/VLS Gains Drv/SLC Tuning/Min Level ==
  TOP : TOP/TOP  TriggerInit=[360 17 565 73]  TopName=MinLevel  DataType=single  BankNumber=0  PreOverlay=false  PostOverlay=false  Role=Automatic
      settings: SourceProductName=Bose Talaria
  TranslateTrigger : TuneVar/TranslateTrigger  TriggerInit=[231 -105 269 -50]
      settings: SourceProductName=Bose Talaria
  Trivial Translation : MATLAB Function  TreatAsAtomicUnit=on
  Tune Variable : TuneVar/TuneVar  TuneName=MinLevel  SpecifyMaxSize=off  VariableDim=1 (Row)  MaxSize=[1 1]  TunabilityNumber=1  MinValue=[0]  MaxValue=[1]  TriggerInit=[-120 20 65 70]  MaskValue=tuneStruct.minGain
      settings: SourceProductName=Bose Talaria
  Out1 : Outport  VectorParamsAs1DForOutWhenUnconnected=off
  wires:
  TranslateTrigger/1 -> Trivial Translation/Trigger
  Trivial Translation/1(TOP) -> TOP/1
  Tune Variable/1 -> Trivial Translation/1(minGain)  "MinLevel"
  TOP/1 -> Out1/1  "MinLevel"

== system VLSGains/VLS Gains Pax/Fade Tuning/Backward Downmix Max ==
  TOP : TOP/TOP  TriggerInit=[440 20 585 80]  TopName=BackwardDownmixMax  DataType=single  BankNumber=0  PreOverlay=false  PostOverlay=false  Role=Automatic
      settings: SourceProductName=Bose Talaria
  TranslateTrigger : TuneVar/TranslateTrigger  TriggerInit=[286 -100 324 -45]
      settings: SourceProductName=Bose Talaria
  Trivial Translation : MATLAB Function  TreatAsAtomicUnit=on
  Tune Variable : TuneVar/TuneVar  TuneName=BackwardDownmixMax  SpecifyMaxSize=off  VariableDim=1 (Row)  MaxSize=[1 1]  TunabilityNumber=1  MinValue=[0]  MaxValue=[1]  TriggerInit=[-65 25 105 75]  MaskValue=tuneStruct.BackwardDownmixMax
      settings: SourceProductName=Bose Talaria
  Out1 : Outport  VectorParamsAs1DForOutWhenUnconnected=off
  wires:
  TranslateTrigger/1 -> Trivial Translation/Trigger
  Trivial Translation/1(TOP) -> TOP/1
  Tune Variable/1 -> Trivial Translation/1(BackwardDownmixMax)  "BackwardDownmixMax"
  TOP/1 -> Out1/1  "BackwardDownmixMax"

== system VLSGains/VLS Gains Pax/Fade Tuning/Backward Downmix Threshold ==
  TOP : TOP/TOP  TriggerInit=[440 20 585 80]  TopName=BackwardDownmixThreshold  DataType=single  BankNumber=0  PreOverlay=false  PostOverlay=false  Role=Automatic
      settings: SourceProductName=Bose Talaria
  TranslateTrigger : TuneVar/TranslateTrigger  TriggerInit=[306 -100 344 -45]
      settings: SourceProductName=Bose Talaria
  Trivial Translation : MATLAB Function  TreatAsAtomicUnit=on
  Tune Variable : TuneVar/TuneVar  TuneName=BackwardDownmixThreshold  SpecifyMaxSize=off  VariableDim=1 (Row)  MaxSize=[1 1]  TunabilityNumber=1  MinValue=[0]  MaxValue=[1]  TriggerInit=[-75 25 95 75]  MaskValue=tuneStruct.BackwardDownmixThreshold
      settings: SourceProductName=Bose Talaria
  Out1 : Outport  VectorParamsAs1DForOutWhenUnconnected=off
  wires:
  TranslateTrigger/1 -> Trivial Translation/Trigger
  Trivial Translation/1(TOP) -> TOP/1
  Tune Variable/1 -> Trivial Translation/1(BackwardDownmixThreshold)  "BackwardDownmixThreshold"
  TOP/1 -> Out1/1  "BackwardDownmixThreshold"

== system VLSGains/VLS Gains Pax/Fade Tuning/Downmix Weights ==
  TOP : TOP/TOP  TriggerInit=[385 17 610 83]  TopName=DownmixWeights  DataType=single  BankNumber=0  PreOverlay=false  PostOverlay=false  Role=Automatic
      settings: SourceProductName=Bose Talaria
  TranslateTrigger : TuneVar/TranslateTrigger  TriggerInit=[266 -100 304 -45]
      settings: SourceProductName=Bose Talaria
  Trivial Translation : MATLAB Function  TreatAsAtomicUnit=on
  Tune Variable : TuneVar/TuneVar  TuneName=DownmixWeights  SpecifyMaxSize=off  VariableDim=1 (Row)  MaxSize=[1 1]  TunabilityNumber=1  MinValue=[0]  MaxValue=[1]  TriggerInit=[-80 25 150 75]  MaskValue=tuneStruct.downmix_wts
      settings: SourceProductName=Bose Talaria
  Out1 : Outport  VectorParamsAs1DForOutWhenUnconnected=off
  wires:
  TranslateTrigger/1 -> Trivial Translation/Trigger
  Trivial Translation/1(TOP) -> TOP/1
  Tune Variable/1 -> Trivial Translation/1(downmix_wts)  "DownmixWeights"
  TOP/1 -> Out1/1  "DownmixWeights"

== system VLSGains/VLS Gains Pax/Fade Tuning/Forward Downmix Threshold ==
  TOP : TOP/TOP  TriggerInit=[440 20 585 80]  TopName=ForwardDownmixThreshold  DataType=single  BankNumber=0  PreOverlay=false  PostOverlay=false  Role=Automatic
      settings: SourceProductName=Bose Talaria
  TranslateTrigger : TuneVar/TranslateTrigger  TriggerInit=[291 -100 329 -45]
      settings: SourceProductName=Bose Talaria
  Trivial Translation : MATLAB Function  TreatAsAtomicUnit=on
  Tune Variable : TuneVar/TuneVar  TuneName=ForwardDownmixThreshold  SpecifyMaxSize=off  VariableDim=1 (Row)  MaxSize=[1 1]  TunabilityNumber=1  MinValue=[0]  MaxValue=[1]  TriggerInit=[-80 25 90 75]  MaskValue=tuneStruct.ForwardDownmixThreshold
      settings: SourceProductName=Bose Talaria
  Out1 : Outport  VectorParamsAs1DForOutWhenUnconnected=off
  wires:
  TranslateTrigger/1 -> Trivial Translation/Trigger
  Trivial Translation/1(TOP) -> TOP/1
  Tune Variable/1 -> Trivial Translation/1(ForwardDownmixThreshold)  "ForwardDownmixThreshold"
  TOP/1 -> Out1/1  "ForwardDownmixThreshold"

== system VLSGains/VLS Gains Pax/Fade Tuning/Foward Downmix Max ==
  TOP : TOP/TOP  TriggerInit=[440 20 585 80]  TopName=ForwardDownmixMax  DataType=single  BankNumber=0  PreOverlay=false  PostOverlay=false  Role=Automatic
      settings: SourceProductName=Bose Talaria
  TranslateTrigger : TuneVar/TranslateTrigger  TriggerInit=[286 -100 324 -45]
      settings: SourceProductName=Bose Talaria
  Trivial Translation : MATLAB Function  TreatAsAtomicUnit=on
  Tune Variable : TuneVar/TuneVar  TuneName=ForwardDownmixMax  SpecifyMaxSize=off  VariableDim=1 (Row)  MaxSize=[1 1]  TunabilityNumber=1  MinValue=[0]  MaxValue=[1]  TriggerInit=[-70 25 100 75]  MaskValue=tuneStruct.ForwardDownmixMax
      settings: SourceProductName=Bose Talaria
  Out1 : Outport  VectorParamsAs1DForOutWhenUnconnected=off
  wires:
  TranslateTrigger/1 -> Trivial Translation/Trigger
  Trivial Translation/1(TOP) -> TOP/1
  Tune Variable/1 -> Trivial Translation/1(ForwardDownmixMax)  "ForwardDownmixMax"
  TOP/1 -> Out1/1  "ForwardDownmixMax"

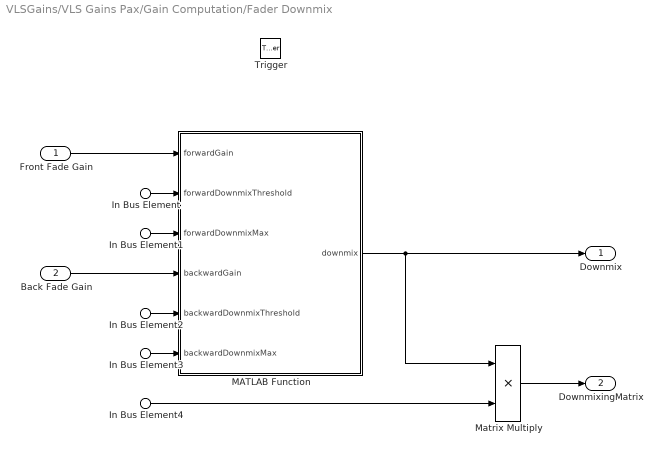
== system VLSGains/VLS Gains Pax/Gain Computation/Fader Downmix ==
  Front Fade Gain : Inport
  Back Fade Gain : Inport  Port=2
  In Bus Element : Inport  Port=3  PortName=Tuned Inputs  Element=Forward Downmix Threshold
  In Bus Element1 : Inport  Port=3  PortName=Tuned Inputs  Element=Forward Downmix Max
  In Bus Element2 : Inport  Port=3  PortName=Tuned Inputs  Element=Backward Downmix Threshold
  In Bus Element3 : Inport  Port=3  PortName=Tuned Inputs  Element=Backward Downmix Max
  In Bus Element4 : Inport  Port=3  PortName=Tuned Inputs  Element=Downmix Weights
  Trigger : TriggerPort  TriggerType=function-call  VariantControl=Variant  PortDimensions=1
  MATLAB Function : MATLAB Function  TreatAsAtomicUnit=on
  Matrix Multiply : Product
  Downmix : Outport  VectorParamsAs1DForOutWhenUnconnected=off
  DownmixingMatrix : Outport  Port=2  VectorParamsAs1DForOutWhenUnconnected=off
  wires:
  In Bus Element4/1 -> Matrix Multiply/2
  Matrix Multiply/1 -> DownmixingMatrix/1
  Back Fade Gain/1 -> MATLAB Function/4(backwardGain)
  Front Fade Gain/1 -> MATLAB Function/1(forwardGain)
  In Bus Element/1 -> MATLAB Function/2(forwardDownmixThreshold)
  In Bus Element1/1 -> MATLAB Function/3(forwardDownmixMax)
  In Bus Element2/1 -> MATLAB Function/5(backwardDownmixThreshold)
  In Bus Element3/1 -> MATLAB Function/6(backwardDownmixMax)
  MATLAB Function/1(downmix) -> Matrix Multiply/1, Downmix/1

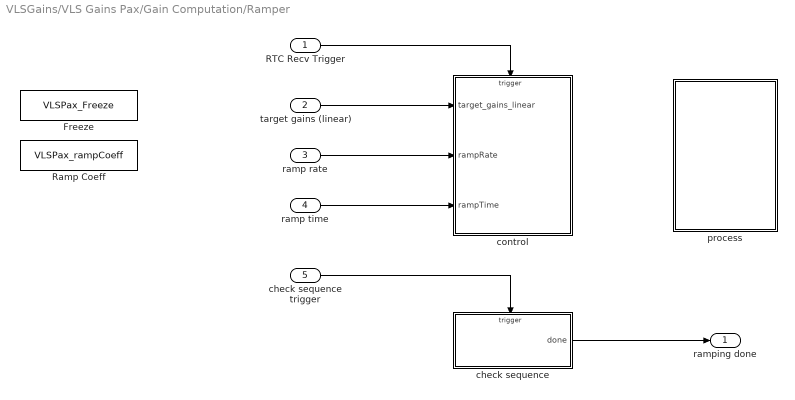
== system VLSGains/VLS Gains Pax/Gain Computation/Ramper ==
  RTC Recv Trigger : Inport
  target gains (linear) : Inport  Port=2
  ramp rate : Inport  Port=3
  ramp time : Inport  Port=4
  check sequence trigger : Inport  Port=5
  Freeze : DataStoreMemory  DataStoreName=VLSPax_Freeze  ReadBeforeWriteMsg=warning  WriteAfterWriteMsg=warning  WriteAfterReadMsg=warning  ShowAdditionalParam=off  OutDataTypeStr=boolean
  Ramp Coeff : DataStoreMemory  DataStoreName=VLSPax_rampCoeff  ReadBeforeWriteMsg=warning  WriteAfterWriteMsg=warning  WriteAfterReadMsg=warning  InitialValue=ones(configStruct.numGains,1)  ShowAdditionalParam=off  OutDataTypeStr=single
  check sequence : MATLAB Function  TreatAsAtomicUnit=on
  control : MATLAB Function  TreatAsAtomicUnit=on
  process : MATLAB Function  TreatAsAtomicUnit=on
  ramping done : Outport  VectorParamsAs1DForOutWhenUnconnected=off
  wires:
  target gains (linear)/1 -> control/1(target_gains_linear)
  RTC Recv Trigger/1 -> control/Trigger
  check sequence/1(done) -> ramping done/1
  check sequence trigger/1 -> check sequence/Trigger
  ramp time/1 -> control/3(rampTime)
  ramp rate/1 -> control/2(rampRate)

== system VLSGains/VLS Gains Pax/Gain Computation/Surround Level Control ==
  RST Trigger : Inport
  SLC Request Trigger : Inport  Port=2
  Surround Index : Inport  Port=3
  In Bus Element3 : Inport  Port=4  PortName=Tuned Inputs  Element=Min Level
  In Bus Element4 : Inport  Port=4  PortName=Tuned Inputs  Element=Detent Level
  In Bus Element5 : Inport  Port=4  PortName=Tuned Inputs  Element=Max Level
  In Bus Element6 : Inport  Port=4  PortName=Tuned Inputs  Element=Interpolation Method
  Data Store Read : DataStoreRead  DataStoreName=VLSPax_SLCGain  IndexOptions=Index vector (dialog)  Indices=1  OutputSizes=1
  Initialization and RMDL : MATLAB Function  TreatAsAtomicUnit=on
  Target Gain Computation : MATLAB Function  TreatAsAtomicUnit=on
  Out1 : Outport
  wires:
  In Bus Element4/1 -> Target Gain Computation/2(detentGain), Initialization and RMDL/2(detentGain)
  In Bus Element3/1 -> Initialization and RMDL/1(minGain), Target Gain Computation/1(minGain)
  In Bus Element6/1 -> Initialization and RMDL/4(interpolation_method), Target Gain Computation/4(interpolation_method)
  In Bus Element5/1 -> Initialization and RMDL/3(maxGain), Target Gain Computation/3(maxGain)
  SLC Request Trigger/1 -> Target Gain Computation/Trigger
  RST Trigger/1 -> Initialization and RMDL/Trigger
  Surround Index/1 -> Initialization and RMDL/5(surr_level), Target Gain Computation/5(surr_level)
  Data Store Read/1 -> Out1/1

== system VLSGains/VLS Gains Pax/SLC Tuning/Detent Level ==
  TOP : TOP/TOP  TriggerInit=[405 22 635 78]  TopName=DetentLevel  DataType=single  BankNumber=0  PreOverlay=false  PostOverlay=false  Role=Automatic
      settings: SourceProductName=Bose Talaria
  TranslateTrigger : TuneVar/TranslateTrigger  TriggerInit=[266 -100 304 -45]
      settings: SourceProductName=Bose Talaria
  Trivial Translation : MATLAB Function  TreatAsAtomicUnit=on
  Tune Variable : TuneVar/TuneVar  TuneName=DetentLevel  SpecifyMaxSize=off  VariableDim=1 (Row)  MaxSize=[1 1]  TunabilityNumber=1  MinValue=[0]  MaxValue=[1]  TriggerInit=[-110 25 105 75]  MaskValue=tuneStruct.detentGain
      settings: SourceProductName=Bose Talaria
  Out1 : Outport  VectorParamsAs1DForOutWhenUnconnected=off
  wires:
  TranslateTrigger/1 -> Trivial Translation/Trigger
  Trivial Translation/1(TOP) -> TOP/1
  Tune Variable/1 -> Trivial Translation/1(detentGain)  "DetentLevel"
  TOP/1 -> Out1/1  "DetentLevel"

== system VLSGains/VLS Gains Pax/SLC Tuning/Interpolation Method ==
  TOP : TOP/TOP  TriggerInit=[440 20 585 80]  TopName=Interpolation_Method  DataType=single  BankNumber=0  PreOverlay=false  PostOverlay=false  Role=Automatic
      settings: SourceProductName=Bose Talaria
  TranslateTrigger : TuneVar/TranslateTrigger  TriggerInit=[306 -100 344 -45]
      settings: SourceProductName=Bose Talaria
  Trivial Translation : MATLAB Function  TreatAsAtomicUnit=on
  Tune Variable : TuneVar/TuneVar  TuneName=Interpolation_Method  SpecifyMaxSize=off  VariableDim=1 (Row)  MaxSize=[1 1]  TunabilityNumber=2  MinValue=[0]  MaxValue=[1]  TriggerInit=[-40 25 130 75]  MaskValue=tuneStruct.interpolationMethod
      settings: SourceProductName=Bose Talaria
  Out1 : Outport  VectorParamsAs1DForOutWhenUnconnected=off
  wires:
  TranslateTrigger/1 -> Trivial Translation/Trigger
  Trivial Translation/1(TOP) -> TOP/1
  Tune Variable/1 -> Trivial Translation/1(interpolationMethod)  "Interpolation_Method"
  TOP/1 -> Out1/1  "Interpolation_Method"

== system VLSGains/VLS Gains Pax/SLC Tuning/Max Level ==
  TOP : TOP/TOP  TriggerInit=[425 22 630 78]  TopName=MaxLevel  DataType=single  BankNumber=0  PreOverlay=false  PostOverlay=false  Role=Automatic
      settings: SourceProductName=Bose Talaria
  TranslateTrigger : TuneVar/TranslateTrigger  TriggerInit=[306 -100 344 -45]
      settings: SourceProductName=Bose Talaria
  Trivial Translation : MATLAB Function  TreatAsAtomicUnit=on
  Tune Variable : TuneVar/TuneVar  TuneName=MaxLevel  SpecifyMaxSize=off  VariableDim=1 (Row)  MaxSize=[1 1]  TunabilityNumber=1  MinValue=[0]  MaxValue=[1]  TriggerInit=[-55 25 145 75]  MaskValue=tuneStruct.maxGain
      settings: SourceProductName=Bose Talaria
  Out1 : Outport  VectorParamsAs1DForOutWhenUnconnected=off
  wires:
  TranslateTrigger/1 -> Trivial Translation/Trigger
  Trivial Translation/1(TOP) -> TOP/1
  Tune Variable/1 -> Trivial Translation/1(maxGain)  "MaxLevel"
  TOP/1 -> Out1/1  "MaxLevel"

== system VLSGains/VLS Gains Pax/SLC Tuning/Min Level ==
  TOP : TOP/TOP  TriggerInit=[360 17 565 73]  TopName=MinLevel  DataType=single  BankNumber=0  PreOverlay=false  PostOverlay=false  Role=Automatic
      settings: SourceProductName=Bose Talaria
  TranslateTrigger : TuneVar/TranslateTrigger  TriggerInit=[231 -105 269 -50]
      settings: SourceProductName=Bose Talaria
  Trivial Translation : MATLAB Function  TreatAsAtomicUnit=on
  Tune Variable : TuneVar/TuneVar  TuneName=MinLevel  SpecifyMaxSize=off  VariableDim=1 (Row)  MaxSize=[1 1]  TunabilityNumber=1  MinValue=[0]  MaxValue=[1]  TriggerInit=[-120 20 65 70]  MaskValue=tuneStruct.minGain
      settings: SourceProductName=Bose Talaria
  Out1 : Outport  VectorParamsAs1DForOutWhenUnconnected=off
  wires:
  TranslateTrigger/1 -> Trivial Translation/Trigger
  Trivial Translation/1(TOP) -> TOP/1
  Tune Variable/1 -> Trivial Translation/1(minGain)  "MinLevel"
  TOP/1 -> Out1/1  "MinLevel"

== matlab function VLSGains/VLS Gains Drv/Fade Tuning/Downmix Weights/Trivial Translation ==
  data: TOP output; downmix_wts input; configStruct parameter
  events: trigger input FUNCTION_CALL_EVENT
function TOP  = fcn(downmix_wts, configStruct)
%#codegen

% Checks if the parameter satisfies dimensionality requirements
if(downmix_wts.Size(1) ~= configStruct.numGains)
    TranslateError('The parameter ''VLS_downmix'' must be a %d element vector.', configStruct.numGains);
end

% Checks if the parameter values follow bound requirements
checkValues = (downmix_wts.Value < 0);
if(sum(sum(checkValues)))          % Results in 0 if all values in the matrix respect the bound requirements
    TranslateError('The weights in ''VLS_downmix'' must be greater than or equal to 0.');
end

TOP = downmix_wts.Value;

end

== matlab function VLSGains/VLS Gains Drv/Fade Tuning/Forward Downmix Threshold/Trivial Translation ==
  data: TOP output; ForwardDownmixThreshold input
  events: trigger input FUNCTION_CALL_EVENT
function TOP  = fcn(ForwardDownmixThreshold)
%#codegen
% Checks if the parameter satisfies dimensionality requirements
if(numel(ForwardDownmixThreshold.Value) ~= 1)
   TranslateError('The parameter ''medusa_forward_downmix_threshold'' must be single dimensional.'); 
end

% Checks if the parameter value follows bound requirements
if((ForwardDownmixThreshold.Value < 0) || (ForwardDownmixThreshold.Value > 1))
   TranslateError('The value of ''medusa_forward_downmix_threshold'' must be between 0 and 1.'); 
end

TOP = ForwardDownmixThreshold.Value;

end

== matlab function VLSGains/VLS Gains Pax/Fade Tuning/Backward Downmix Threshold/Trivial Translation ==
  data: TOP output; BackwardDownmixThreshold input
  events: trigger input FUNCTION_CALL_EVENT
function TOP  = fcn(BackwardDownmixThreshold)
%#codegen
% Checks if the parameter satisfies dimensionality requirements
if(numel(BackwardDownmixThreshold.Value) ~= 1)
   TranslateError('The parameter ''medusa_backward_downmix_threshold'' must be single dimensional.'); 
end

% Checks if the parameter value follows bound requirements
if((BackwardDownmixThreshold.Value < 0) || (BackwardDownmixThreshold.Value > 1))
   TranslateError('The value of ''medusa_backward_downmix_threshold'' must be between 0 and 1.'); 
end

TOP = BackwardDownmixThreshold.Value;

end

== matlab function VLSGains/VLS Gains Drv/Fade Tuning/Foward Downmix Max/Trivial Translation ==
  data: TOP output; ForwardDownmixMax input
  events: trigger input FUNCTION_CALL_EVENT
function TOP  = fcn(ForwardDownmixMax)
%#codegen
% Checks if the parameter satisfies dimensionality requirements
if(numel(ForwardDownmixMax.Value) ~= 1)
   TranslateError('The parameter ''medusa_forward_downmix_max'' must be single dimensional.'); 
end

% Checks if the parameter value follows bound requirements
if((ForwardDownmixMax.Value < 0) || (ForwardDownmixMax.Value > 1))
   TranslateError('The value of ''medusa_forward_downmix_max'' must be between 0 and 1.'); 
end

TOP = ForwardDownmixMax.Value;

end

== matlab function VLSGains/VLS Gains Pax/Fade Tuning/Downmix Weights/Trivial Translation ==
  data: TOP output; downmix_wts input; configStruct parameter
  events: trigger input FUNCTION_CALL_EVENT
function TOP  = fcn(downmix_wts, configStruct)
%#codegen

% Checks if the parameter satisfies dimensionality requirements
if(downmix_wts.Size(1) ~= configStruct.numGains)
    TranslateError('The parameter ''VLS_downmix'' must be a %d element vector.', configStruct.numGains);
end

% Checks if the parameter values follow bound requirements
checkValues = (downmix_wts.Value < 0);
if(sum(sum(checkValues)))          % Results in 0 if all values in the matrix respect the bound requirements
    TranslateError('The weights in ''VLS_downmix'' must be greater than or equal to 0.');
end

TOP = downmix_wts.Value;

end
